simulink model "llmse"  (R2021a)
settings: Solver=VariableStepAuto  StartTime=0.0  StopTime=10.0  RelTol=1e-3
values from neighbouring files (symbols this model uses):
  DT = 1.0    (= 1)    [runllmse.m]
  H = [0.1685   -0.9595   -0.0755   -0.3771 ... (first row only)    [runkalmanfilter.m]    (also in runllmse.m = randn(N,4))
  M_AP = eye(4)    [runllmse.m]
  sigma_n = 0.5    [runllmse.m]
  theta_AP = zeros(4,1)    [runllmse.m]
  x = H*theta + W    [runllmse.m]
settings Model: Creator=j21lys  LastModifiedBy=j21lys

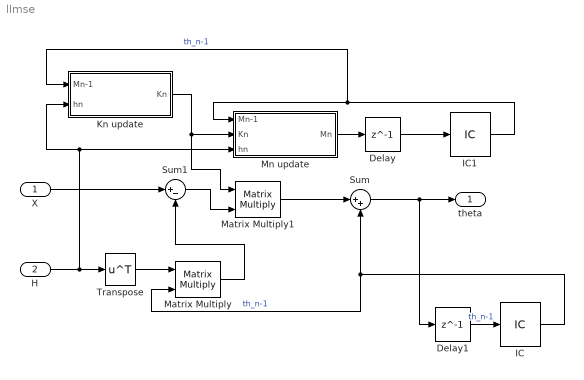
== system llmse ==
  X : Inport  PortDimensions=size(x, 2)
  H : Inport  Port=2  PortDimensions=size(H, 2)
  Delay : Delay  DelayLength=1  InitialCondition=0
  Delay1 : Delay  DelayLength=1  InitialCondition=0
  IC : InitialCondition  Value=theta_AP
  IC1 : InitialCondition  Value=M_AP
  Kn update : Subsystem
  Matrix Multiply : Product  Multiplication=Matrix(*)
  Matrix Multiply1 : Product  Multiplication=Matrix(*)
  Mn update : Subsystem
  Sum : Sum  Inputs=|++
  Sum1 : Sum  Inputs=|+-
  Transpose : Math  Operator=transpose  SaturateOnIntegerOverflow=on
  theta : Outport  SampleTime=DT
  wires:
  Mn update/1(Mn) -> Delay/1
  Kn update/1(Kn) -> Matrix Multiply1/1, Mn update/2(Kn)
  Sum/1 -> Delay1/1, theta/1
  IC/1 -> Sum/2, Matrix Multiply/2  "th_n-1"
  H/1 -> Kn update/2(hn), Mn update/3(hn), Transpose/1
  Transpose/1 -> Matrix Multiply/1
  Matrix Multiply/1 -> Sum1/2
  X/1 -> Sum1/1
  Sum1/1 -> Matrix Multiply1/2
  Matrix Multiply1/1 -> Sum/1
  Delay1/1 -> IC/1  "th_n-1"
  Delay/1 -> IC1/1
  IC1/1 -> Kn update/1(Mn-1), Mn update/1(Mn-1)  "th_n-1"

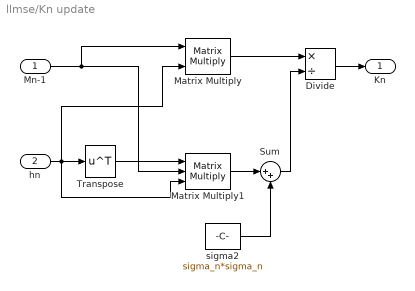
== system llmse/Kn update ==
  Mn-1 : Inport
  hn : Inport  Port=2
  Divide : Product  Inputs=*/
  Matrix Multiply : Product  Multiplication=Matrix(*)
  Matrix Multiply1 : Product  Inputs=3  Multiplication=Matrix(*)
  Sum : Sum  Inputs=|++
  Transpose : Math  Operator=transpose  SaturateOnIntegerOverflow=on
  sigma2 : Constant  Value=sigma_n*sigma_n
  Kn : Outport
  wires:
  hn/1 -> Matrix Multiply/2, Matrix Multiply1/3, Transpose/1
  Transpose/1 -> Matrix Multiply1/1
  Mn-1/1 -> Matrix Multiply/1, Matrix Multiply1/2
  Matrix Multiply1/1 -> Sum/1
  sigma2/1 -> Sum/2
  Matrix Multiply/1 -> Divide/1
  Sum/1 -> Divide/2
  Divide/1 -> Kn/1

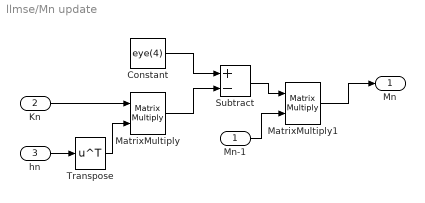
== system llmse/Mn update ==
  Mn-1 : Inport
  Kn : Inport  Port=2
  hn : Inport  Port=3
  Constant : Constant  Value=eye(4)
  MatrixMultiply : Product  Multiplication=Matrix(*)
  MatrixMultiply1 : Product  Multiplication=Matrix(*)
  Subtract : Sum  Inputs=+-
  Transpose : Math  Operator=transpose  SaturateOnIntegerOverflow=on
  Mn : Outport
  wires:
  Kn/1 -> MatrixMultiply/1
  hn/1 -> Transpose/1
  Transpose/1 -> MatrixMultiply/2
  Constant/1 -> Subtract/1
  MatrixMultiply/1 -> Subtract/2
  Subtract/1 -> MatrixMultiply1/1
  Mn-1/1 -> MatrixMultiply1/2
  MatrixMultiply1/1 -> Mn/1
